simulink model "Hp_com"  (R2022b)
settings: Solver=FixedStepAuto  StartTime=0.0  StopTime=10.0  RelTol=1e-3
libraries: simulink x3
settings Model: Creator=86134  LastModifiedBy=86134

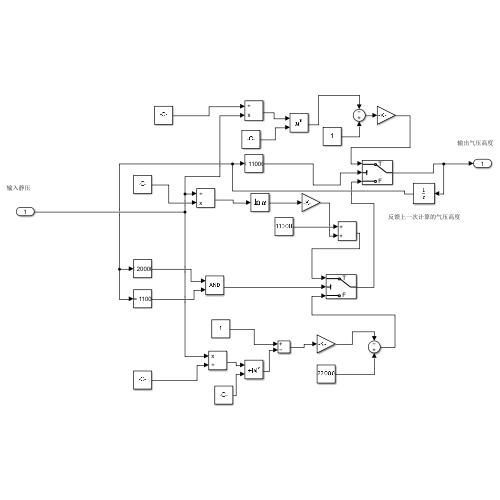
[thumbnail: Simulink's stored preview of the top-level diagram]
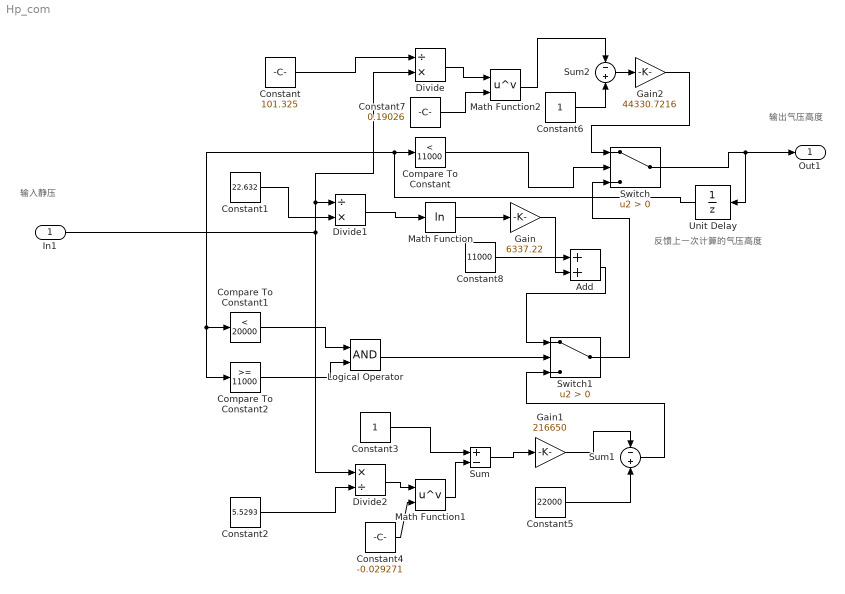
== system Hp_com ==
  note: 反馈上一次计算的气压高度
  note: 输出气压高度
  note: 输入静压
  In1 : Inport
  Add : Sum
  Compare To Constant : simulink/Logic and Bit Operations/Compare To Constant  relop=<  const=11000  OutDataTypeStr=boolean
  Compare To Constant1 : simulink/Logic and Bit Operations/Compare To Constant  relop=<  const=20000  OutDataTypeStr=boolean
  Compare To Constant2 : simulink/Logic and Bit Operations/Compare To Constant  relop=>=  const=11000  OutDataTypeStr=boolean
  Constant : Constant  Value=101.325
  Constant1 : Constant  Value=22.632
  Constant2 : Constant  Value=5.5293
  Constant3 : Constant
  Constant4 : Constant  Value=-0.029271
  Constant5 : Constant  Value=22000
  Constant6 : Constant
  Constant7 : Constant  Value=0.19026
  Constant8 : Constant  Value=11000
  Divide : Product  Inputs=/*
  Divide1 : Product  Inputs=/*
  Divide2 : Product  Inputs=*/
  Gain : Gain  Gain=6337.22
  Gain1 : Gain  Gain=216650
  Gain2 : Gain  Gain=44330.7216
  Logical Operator : Logic  AllPortsSameDT=off  OutDataTypeStr=boolean
  Math Function : Math  Operator=log
  Math Function1 : Math  Operator=pow  SignedPower=on
  Math Function2 : Math  Operator=pow
  Sum : Sum  Inputs=+-
  Sum1 : Sum  Inputs=-+
  Sum2 : Sum  Inputs=-+
  Switch : Switch  Criteria=u2 > Threshold  SaturateOnIntegerOverflow=off  InputSameDT=off
  Switch1 : Switch  Criteria=u2 > Threshold  SaturateOnIntegerOverflow=off  InputSameDT=off
  Unit Delay : UnitDelay  SampleTime=-1  HasFrameUpgradeWarning=on
  Out1 : Outport
  wires:
  Compare To Constant/1 -> Switch/2
  In1/1 -> Divide/2, Divide1/1, Divide2/1
  Constant/1 -> Divide/1
  Compare To Constant1/1 -> Logical Operator/1
  Compare To Constant2/1 -> Logical Operator/2
  Logical Operator/1 -> Switch1/2
  Constant1/1 -> Divide1/2
  Divide1/1 -> Math Function/1
  Math Function/1 -> Gain/1
  Gain/1 -> Add/2
  Add/1 -> Switch1/1
  Constant2/1 -> Divide2/2
  Constant3/1 -> Sum/1
  Divide2/1 -> Math Function1/1
  Constant4/1 -> Math Function1/2
  Math Function1/1 -> Sum/2
  Sum/1 -> Gain1/1
  Gain1/1 -> Sum1/1
  Constant5/1 -> Sum1/2
  Sum1/1 -> Switch1/3
  Switch1/1 -> Switch/3
  Switch/1 -> Unit Delay/1, Out1/1
  Constant6/1 -> Sum2/2
  Divide/1 -> Math Function2/1
  Constant7/1 -> Math Function2/2
  Math Function2/1 -> Sum2/1
  Sum2/1 -> Gain2/1
  Gain2/1 -> Switch/1
  Unit Delay/1 -> Compare To Constant2/1, Compare To Constant1/1, Compare To Constant/1
  Constant8/1 -> Add/1
